simulink model "EVSystemConverterModel"  (R2024a)
settings: Solver=ode23t  StartTime=0.0  StopTime=0.08  RelTol=1e-3
libraries: fl_lib x16, nesl_utility x8, ee_lib x3, eePwmGenerator x3, batteryecm_lib x1
settings Model: Creator=callie  LastModifiedBy=callie
settings DataIOCC: ReturnWorkspaceOutputs=off
settings SimscapeCC: SimscapeLogType=all  SimscapeLogLimitData=off

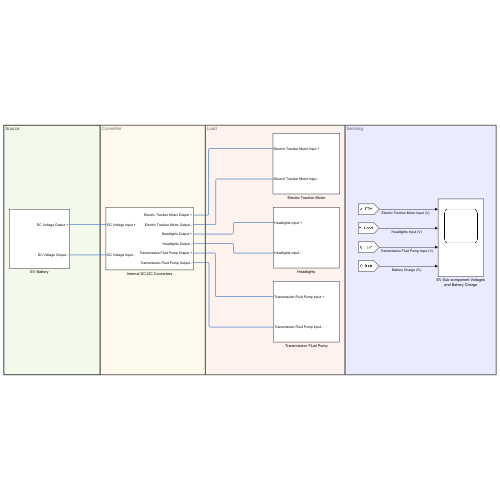
[thumbnail: Simulink's stored preview of the top-level diagram]
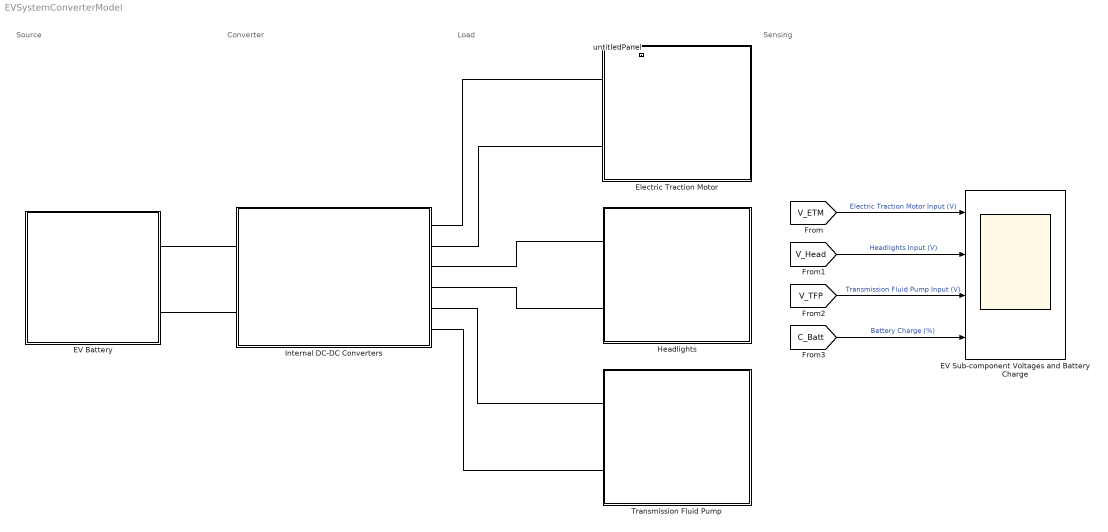
== system EVSystemConverterModel ==
  note: Sensing
  note: Load
  note: Converter
  note: Source
  EV Battery : Subsystem
      settings: PortSchema="{\"entries\":[{\"content\":{\"sides\":[{\"content\":{},\"type\":\"ConnectorPlacement.EquallySpacedRectSide\",\"uuid\":\"c6623932-9384-4505-9c8a-7aa7c6d03efe\"},{\"content\":{\"side\":\"RIGHT\"},\"type\":\"ConnectorPlacement.EquallySpacedRectSide\",\"uuid\":\"b63081fa-6f2e-4d52-89b7-0b15c2ff5a8a\"},{\"content\":{\"side\":\"TOP\"},\"type\":\"ConnectorPlacement.EquallySpacedRectSide\",\"uuid\":\"293a2b80-333e-46a9-baf9-140dd0ae167b\"},{\"content\":{\"connectorIds\":[\"RConn1\",\"RConn2\"],\"side\":\"BOTTOM\"},\"type\":\"ConnectorPlacement.EquallySpacedRectSide\",\"uuid\":\"5c4d294a-cecf-4357-a6de-56f8bde29aff\"}]},\"type\":\"ConnectorPlacement.EquallySpacedConnector\",\"uuid\":\"b1957f8b-46fc-490a-ae52-971fc17beee3\"}],\"packageUris\":[\"http://schema.mathworks.com/mf0/Connector/R2020b\"],\"version\":\"1.0\"}"
  EV Sub-component Voltages and Battery Charge : Scope  NumInputPorts=4
  Electric Traction Motor : Subsystem
      settings: PortSchema="{\"entries\":[{\"content\":{\"sides\":[{\"content\":{},\"type\":\"ConnectorPlacement.EquallySpacedRectSide\",\"uuid\":\"1c916003-081d-495c-ab06-e1419b6c539b\"},{\"content\":{\"side\":\"RIGHT\"},\"type\":\"ConnectorPlacement.EquallySpacedRectSide\",\"uuid\":\"f192687e-cae6-4b69-b15b-4d7b02c42b9f\"},{\"content\":{\"connectorIds\":[\"LConn1\",\"LConn2\"],\"side\":\"TOP\"},\"type\":\"ConnectorPlacement.EquallySpacedRectSide\",\"uuid\":\"4ee18eaf-a0eb-4206-a34f-c6cf4701fcf7\"}]},\"type\":\"ConnectorPlacement.EquallySpacedConnector\",\"uuid\":\"c4b359e2-4be8-4ef0-b2fa-d43323f3e4c6\"}],\"packageUris\":[\"http://schema.mathworks.com/mf0/Connector/R2020b\"],\"version\":\"1.0\"}"
  Headlights : Subsystem
      settings: PortSchema="{\"entries\":[{\"content\":{\"sides\":[{\"content\":{},\"type\":\"ConnectorPlacement.EquallySpacedRectSide\",\"uuid\":\"1c916003-081d-495c-ab06-e1419b6c539b\"},{\"content\":{\"side\":\"RIGHT\"},\"type\":\"ConnectorPlacement.EquallySpacedRectSide\",\"uuid\":\"f192687e-cae6-4b69-b15b-4d7b02c42b9f\"},{\"content\":{\"connectorIds\":[\"LConn1\",\"LConn2\"],\"side\":\"TOP\"},\"type\":\"ConnectorPlacement.EquallySpacedRectSide\",\"uuid\":\"4ee18eaf-a0eb-4206-a34f-c6cf4701fcf7\"}]},\"type\":\"ConnectorPlacement.EquallySpacedConnector\",\"uuid\":\"c4b359e2-4be8-4ef0-b2fa-d43323f3e4c6\"}],\"packageUris\":[\"http://schema.mathworks.com/mf0/Connector/R2020b\"],\"version\":\"1.0\"}"
  Internal DC-DC Converters : Subsystem
  Transmission Fluid Pump : Subsystem
      settings: PortSchema="{\"entries\":[{\"content\":{\"sides\":[{\"content\":{},\"type\":\"ConnectorPlacement.EquallySpacedRectSide\",\"uuid\":\"1c916003-081d-495c-ab06-e1419b6c539b\"},{\"content\":{\"side\":\"RIGHT\"},\"type\":\"ConnectorPlacement.EquallySpacedRectSide\",\"uuid\":\"f192687e-cae6-4b69-b15b-4d7b02c42b9f\"},{\"content\":{\"connectorIds\":[\"LConn1\",\"LConn2\"],\"side\":\"TOP\"},\"type\":\"ConnectorPlacement.EquallySpacedRectSide\",\"uuid\":\"4ee18eaf-a0eb-4206-a34f-c6cf4701fcf7\"}]},\"type\":\"ConnectorPlacement.EquallySpacedConnector\",\"uuid\":\"c4b359e2-4be8-4ef0-b2fa-d43323f3e4c6\"}],\"packageUris\":[\"http://schema.mathworks.com/mf0/Connector/R2020b\"],\"version\":\"1.0\"}"
  untitledPanel : Subsystem  Tag=HiddenForWebPanel  IsWebBlockPanel=on
  wires:
  [V_TFP] -> EV Sub-component Voltages and Battery Charge/3  "Transmission Fluid Pump Input (V)"
  [C_Batt] -> EV Sub-component Voltages and Battery Charge/4  "Battery Charge (%)"
  [V_Head] -> EV Sub-component Voltages and Battery Charge/2  "Headlights Input (V)"
  [V_ETM] -> EV Sub-component Voltages and Battery Charge/1  "Electric Traction Motor Input (V)"
  connections:
  EV Battery/RConn1 -- Internal DC-DC Converters/RConn1
  EV Battery/RConn2 -- Internal DC-DC Converters/RConn2
  Internal DC-DC Converters/LConn1 -- Electric Traction Motor/LConn1
  Internal DC-DC Converters/LConn2 -- Electric Traction Motor/LConn2
  Internal DC-DC Converters/LConn3 -- Headlights/LConn1
  Internal DC-DC Converters/LConn4 -- Headlights/LConn2
  Internal DC-DC Converters/LConn5 -- Transmission Fluid Pump/LConn1
  Transmission Fluid Pump/LConn2 -- Internal DC-DC Converters/LConn6

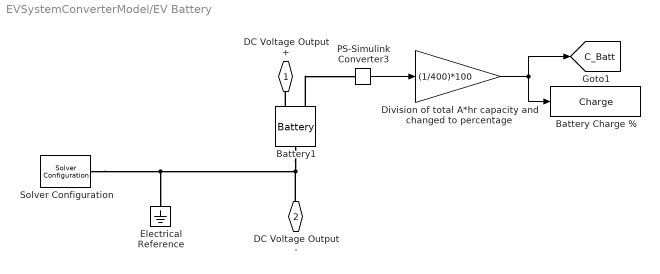
== system EVSystemConverterModel/EV Battery ==
  Battery Charge % : ToWorkspace  VariableName=Charge  SampleTime=-1
  Battery1 : batteryecm_lib/Battery  Vnom=350 V  prm_dir=simscape.enum.battery.prm_dir.disabled  R1_dis=2 Ohm  R1_ch=2 Ohm  R1=500 mOhm  prm_AH=simscape.enum.battery.prm_AH.finite  AH=400 A*hr  V1=290 V  AH1=331 A*hr  prm_R2=simscape.enum.battery.prm_R2.disabled  R2=2000 Ohm  Tmeas=298.15 K  charge_measurement_port=simscape.enum.battery.enable.yes  prm_dyn=simscape.enum.battery.prm_dyn.off  Rp1=0.005 Ohm  tau1=30 s  Rp2=0.005 Ohm  tau2=30 s  Rp3=0.005 Ohm  tau3=30 s  Rp4=0.005 Ohm  tau4=30 s  Rp5=0.005 Ohm  tau5=30 s  prm_fade=simscape.enum.battery.prm_fade.disabled  N_fade=100  AH_fade=45 A*hr  R1_fade=2.02 Ohm  R1_ch_fade=2.02 Ohm  V1_fade=10.35 V  prm_age=simscape.enum.battery.prm_age.disabled  prm_age_OCV=simscape.enum.battery.prm_age_OCV.OCV  OCV_age=0.9  SOC_age=60  Tmeas_age=298.15 K  delta_time_age_vec=[0] d  temperature_age_vec=[273] K  OCV_scaling_age=2.2134e6  OCV_offset_age=1.632e6  temp_exp_age=0.515833569 V  t_exp_age=0.75  Vnom_T2=12 V  R1_T2=2.2 Ohm  R1_T2_dis=2.2 Ohm  R1_T2_ch=2.2 Ohm  V1_T2=11.4 V  R2_T2=2200 Ohm  Rp1_T2=0.005 Ohm  tau1_T2=30 s  Rp2_T2=0.005 Ohm  tau2_T2=30 s  Rp3_T2=0.005 Ohm  tau3_T2=30 s  Rp4_T2=0.005 Ohm  tau4_T2=30 s  Rp5_T2=0.005 Ohm  tau5_T2=30 s  Tmeas2=273.15 K  thermal_port=simscape.enum.thermaleffects.omit  thermal_mass=30000 J/K  i_specify=off  i_priority=None  i=0 A  i_nominal_specify=off  i_nominal_value=1  i_nominal_unit=A  v_specify=on  v_priority=None  v=350 V  v_nominal_specify=off  v_nominal_value=22.8  v_nominal_unit=V  charge_specify=on  charge_priority=High  charge=400 A*hr  charge_nominal_specify=on  charge_nominal_value=2.3  charge_nominal_unit=A*hr  num_cycles_specify=off  num_cycles_priority=High  num_cycles=0  num_cycles_nominal_specify=off  num_cycles_nominal_value=1  num_cycles_nominal_unit=1  temperature_specify=off  temperature_priority=High  temperature=298.15 K  temperature_nominal_specify=off  temperature_nominal_value=1  temperature_nominal_unit=K
      settings: LibrarySourceBlock=batt_lib/Cells/Battery  InternalSimscapePortConfiguration="{\"Bottom\":[],\"Left\":[{\"id\":\"p\",\"label\":\"+\",\"type\":\"foundation.electrical.electrical\"},{\"id\":\"q\",\"label\":\"q\",\"type\":\"output\"}],\"Right\":[{\"id\":\"n\",\"label\":\"-\",\"type\":\"foundation.electrical.electrical\"}],\"Top\":[]}"
  Division of total A*hr capacity and changed to percentage : Gain  Gain=(1/400)*100
  Electrical Reference : fl_lib/Electrical/Electrical Elements/Electrical Reference
  PS-Simulink Converter3 : nesl_utility/PS-Simulink Converter  PhysicalDomain=network_engine_domain  SubClassName=ps_output  LeftPortType=input  RightPortType=output  PseudoPeriodic=off  Frequencies=[]  VectorFormat=inherit  Unit=A*hr  AffineConversion=off
  Solver Configuration : nesl_utility/Solver Configuration  PhysicalDomain=network_engine_domain  SubClassName=solver  LeftPortType=input  RightPortType=generic  Tones=[]  Harmonics=[]  SimulateNoise=off  Profile=off  UseLocalSampling=off  EnableSwitchedLinearOptims=on  FrequencyDomain=off  UseCCode=off  RelTol=0.001  AbsTol=1e-06  MinStep=1e-09  ToWorkspace=off  RevertToSquareIcSolve=off  NumHomotopyIterations=100  PhasorMode=off  PhasorModeNumHarmonics=1  ConsistencySolver=NEWTON_FTOL  IndexReductionMethod=DerivativeReplacement  DoDC=off  ResidualTolerance=1e-09  ConsistencyTolSource=GLOBAL  ConsistencyAbsTol=0.001  ConsistencyRelTol=0.001  ConsistencyTolFactor=0.001  UseLocalSolver=off  LocalSolverChoice=NE_BACKWARD_EULER_ADVANCER  ResolveIndetEquations=on  FunctionEvalNumThread=1  LocalSolverSampleTime=0.00001  DoFixedCost=off  MaxNonlinIter=3  MaxModeIter=2  ComputeImpulses=off  ImpulseIterations=2  LinearAlgebra=auto  LinearAlgebraNumThread=0  EquationFormulation=NE_TIME_EF  DelaysMemoryBudget=1024  AutomaticFiltering=on  FilteringTimeConstant=0.001  PartitionStorageMethod=AS_NEEDED  PartitionMemoryBudget=1024  PartitionMethod=ROBUST  MultibodyUseLocalSolver=off  MultibodyLocalSolverChoice=ODE1  MultibodyLocalSolverSampleTime=0.001
  DC Voltage Output + : PMIOPort  Side=Right
  DC Voltage Output - : PMIOPort  Port=2  Side=Right
  tag scope: C_Batt=global
  wires:
  Division of total A*hr capacity and changed to percentage/1 -> [C_Batt], Battery Charge %/1
  PS-Simulink Converter3/1 -> Division of total A*hr capacity and changed to percentage/1
  connections:
  Solver Configuration/RConn1 -- Battery1/RConn1 -- DC Voltage Output -/RConn1 -- Electrical Reference/LConn1
  Battery1/LConn1 -- DC Voltage Output +/RConn1
  Battery1/LConn2 -- PS-Simulink Converter3/LConn1

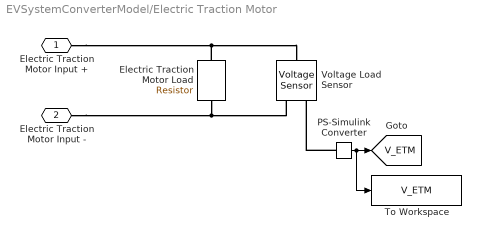
== system EVSystemConverterModel/Electric Traction Motor ==
  Electric Traction Motor Load : fl_lib/Electrical/Electrical Elements/Resistor  R=3 Ohm  i_specify=off  i_priority=High  i=0 A  i_nominal_specify=off  i_nominal_value=1  i_nominal_unit=A  v_specify=off  v_priority=High  v=0 V  v_nominal_specify=off  v_nominal_value=1  v_nominal_unit=V
  PS-Simulink Converter : nesl_utility/PS-Simulink Converter  PhysicalDomain=network_engine_domain  SubClassName=ps_output  LeftPortType=input  RightPortType=output  PseudoPeriodic=off  Frequencies=[]  VectorFormat=inherit  Unit=V  AffineConversion=off
  To Workspace : ToWorkspace  VariableName=V_ETM  SampleTime=-1
  Voltage Load Sensor : fl_lib/Electrical/Electrical Sensors/Voltage Sensor
  Electric Traction Motor Input + : PMIOPort  Side=Left
  Electric Traction Motor Input - : PMIOPort  Port=2  Side=Left
  tag scope: V_ETM=global
  wires:
  PS-Simulink Converter/1 -> To Workspace/1, [V_ETM]
  connections:
  Electric Traction Motor Input -/RConn1 -- Electric Traction Motor Load/RConn1 -- Voltage Load Sensor/RConn2
  Electric Traction Motor Input +/RConn1 -- Electric Traction Motor Load/LConn1 -- Voltage Load Sensor/LConn1
  PS-Simulink Converter/LConn1 -- Voltage Load Sensor/RConn1

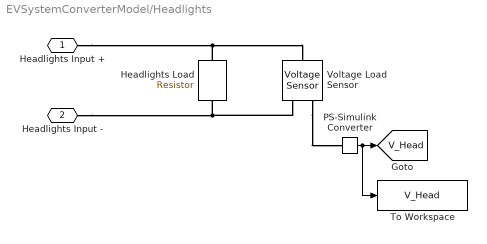
== system EVSystemConverterModel/Headlights ==
  Headlights Load : fl_lib/Electrical/Electrical Elements/Resistor  R=20 Ohm  i_specify=off  i_priority=High  i=0 A  i_nominal_specify=off  i_nominal_value=1  i_nominal_unit=A  v_specify=off  v_priority=High  v=0 V  v_nominal_specify=off  v_nominal_value=1  v_nominal_unit=V
  PS-Simulink Converter : nesl_utility/PS-Simulink Converter  PhysicalDomain=network_engine_domain  SubClassName=ps_output  LeftPortType=input  RightPortType=output  PseudoPeriodic=off  Frequencies=[]  VectorFormat=inherit  Unit=V  AffineConversion=off
  To Workspace : ToWorkspace  VariableName=V_Head  SampleTime=-1
  Voltage Load Sensor : fl_lib/Electrical/Electrical Sensors/Voltage Sensor
  Headlights Input + : PMIOPort  Side=Left
  Headlights Input - : PMIOPort  Port=2  Side=Left
  tag scope: V_Head=global
  wires:
  PS-Simulink Converter/1 -> To Workspace/1, [V_Head]
  connections:
  Headlights Load/LConn1 -- Headlights Input +/RConn1 -- Voltage Load Sensor/LConn1
  Voltage Load Sensor/RConn2 -- Headlights Input -/RConn1 -- Headlights Load/RConn1
  Voltage Load Sensor/RConn1 -- PS-Simulink Converter/LConn1

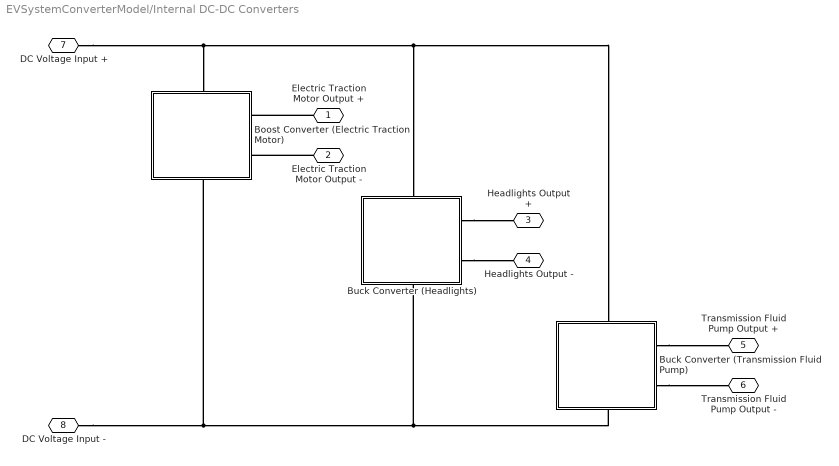
== system EVSystemConverterModel/Internal DC-DC Converters ==
  "Boost Converter (Electric Traction Motor)  " : Subsystem
      settings: PortSchema="{\"entries\":[{\"content\":{\"sides\":[{\"content\":{},\"type\":\"ConnectorPlacement.EquallySpacedRectSide\",\"uuid\":\"de7f9f94-85d7-4c11-a379-f82d9a676ef7\"},{\"content\":{\"connectorIds\":[\"RConn1\",\"RConn2\"],\"side\":\"RIGHT\"},\"type\":\"ConnectorPlacement.EquallySpacedRectSide\",\"uuid\":\"401d076f-92b5-441a-942d-9f536a3912de\"},{\"content\":{\"connectorIds\":[\"LConn1\"],\"side\":\"TOP\"},\"type\":\"ConnectorPlacement.EquallySpacedRectSide\",\"uuid\":\"060ca2a1-5903-409e-b252-71c13fd12de7\"},{\"content\":{\"connectorIds\":[\"RConn3\"],\"side\":\"BOTTOM\"},\"type\":\"ConnectorPlacement.EquallySpacedRectSide\",\"uuid\":\"bdbe130f-4b5d-4c03-bda1-a69c86499370\"}]},\"type\":\"ConnectorPlacement.EquallySpacedConnector\",\"uuid\":\"c546e283-911b-4991-8697-f1e295eb6532\"}],\"packageUris\":[\"http://schema.mathworks.com/mf0/Connector/R2020b\"],\"version\":\"1.0\"}"
  "Buck Converter (Transmission Fluid Pump)  " : Subsystem
      settings: PortSchema="{\"entries\":[{\"content\":{\"sides\":[{\"content\":{},\"type\":\"ConnectorPlacement.EquallySpacedRectSide\",\"uuid\":\"de7f9f94-85d7-4c11-a379-f82d9a676ef7\"},{\"content\":{\"connectorIds\":[\"RConn1\",\"RConn2\"],\"side\":\"RIGHT\"},\"type\":\"ConnectorPlacement.EquallySpacedRectSide\",\"uuid\":\"401d076f-92b5-441a-942d-9f536a3912de\"},{\"content\":{\"connectorIds\":[\"LConn1\"],\"side\":\"TOP\"},\"type\":\"ConnectorPlacement.EquallySpacedRectSide\",\"uuid\":\"060ca2a1-5903-409e-b252-71c13fd12de7\"},{\"content\":{\"connectorIds\":[\"RConn3\"],\"side\":\"BOTTOM\"},\"type\":\"ConnectorPlacement.EquallySpacedRectSide\",\"uuid\":\"bdbe130f-4b5d-4c03-bda1-a69c86499370\"}]},\"type\":\"ConnectorPlacement.EquallySpacedConnector\",\"uuid\":\"c546e283-911b-4991-8697-f1e295eb6532\"}],\"packageUris\":[\"http://schema.mathworks.com/mf0/Connector/R2020b\"],\"version\":\"1.0\"}"
  "Buck Converter (Headlights)  " : Subsystem
      settings: PortSchema="{\"entries\":[{\"content\":{\"sides\":[{\"content\":{},\"type\":\"ConnectorPlacement.EquallySpacedRectSide\",\"uuid\":\"de7f9f94-85d7-4c11-a379-f82d9a676ef7\"},{\"content\":{\"connectorIds\":[\"RConn1\",\"RConn2\"],\"side\":\"RIGHT\"},\"type\":\"ConnectorPlacement.EquallySpacedRectSide\",\"uuid\":\"401d076f-92b5-441a-942d-9f536a3912de\"},{\"content\":{\"connectorIds\":[\"LConn1\"],\"side\":\"TOP\"},\"type\":\"ConnectorPlacement.EquallySpacedRectSide\",\"uuid\":\"060ca2a1-5903-409e-b252-71c13fd12de7\"},{\"content\":{\"connectorIds\":[\"RConn3\"],\"side\":\"BOTTOM\"},\"type\":\"ConnectorPlacement.EquallySpacedRectSide\",\"uuid\":\"bdbe130f-4b5d-4c03-bda1-a69c86499370\"}]},\"type\":\"ConnectorPlacement.EquallySpacedConnector\",\"uuid\":\"c546e283-911b-4991-8697-f1e295eb6532\"}],\"packageUris\":[\"http://schema.mathworks.com/mf0/Connector/R2020b\"],\"version\":\"1.0\"}"
  Electric Traction Motor Output + : PMIOPort  Side=Left
  Electric Traction Motor Output - : PMIOPort  Port=2  Side=Left
  Headlights Output + : PMIOPort  Port=3  Side=Left
  Headlights Output - : PMIOPort  Port=4  Side=Left
  Transmission Fluid Pump Output + : PMIOPort  Port=5  Side=Left
  Transmission Fluid Pump Output - : PMIOPort  Port=6  Side=Left
  DC Voltage Input + : PMIOPort  Port=7  Side=Right
  DC Voltage Input - : PMIOPort  Port=8  Side=Right
  connections:
  DC Voltage Input +/RConn1 -- "Buck Converter (Transmission Fluid Pump)  "/LConn1 -- "Buck Converter (Headlights)  "/LConn1 -- "Boost Converter (Electric Traction Motor)  "/LConn1
  DC Voltage Input -/RConn1 -- "Boost Converter (Electric Traction Motor)  "/RConn3 -- "Buck Converter (Transmission Fluid Pump)  "/RConn3 -- "Buck Converter (Headlights)  "/RConn3
  Electric Traction Motor Output +/RConn1 -- "Boost Converter (Electric Traction Motor)  "/RConn1
  Electric Traction Motor Output -/RConn1 -- "Boost Converter (Electric Traction Motor)  "/RConn2
  "Buck Converter (Headlights)  "/RConn1 -- Headlights Output +/RConn1
  "Buck Converter (Headlights)  "/RConn2 -- Headlights Output -/RConn1
  "Buck Converter (Transmission Fluid Pump)  "/RConn1 -- Transmission Fluid Pump Output +/RConn1
  "Buck Converter (Transmission Fluid Pump)  "/RConn2 -- Transmission Fluid Pump Output -/RConn1

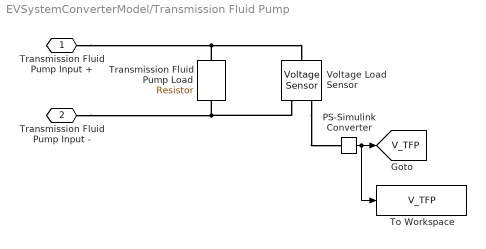
== system EVSystemConverterModel/Transmission Fluid Pump ==
  PS-Simulink Converter : nesl_utility/PS-Simulink Converter  PhysicalDomain=network_engine_domain  SubClassName=ps_output  LeftPortType=input  RightPortType=output  PseudoPeriodic=off  Frequencies=[]  VectorFormat=inherit  Unit=V  AffineConversion=off
  To Workspace : ToWorkspace  VariableName=V_TFP  SampleTime=-1
  Transmission Fluid Pump Load : fl_lib/Electrical/Electrical Elements/Resistor  R=40 Ohm  i_specify=off  i_priority=High  i=0 A  i_nominal_specify=off  i_nominal_value=1  i_nominal_unit=A  v_specify=off  v_priority=High  v=0 V  v_nominal_specify=off  v_nominal_value=1  v_nominal_unit=V
  Voltage Load Sensor : fl_lib/Electrical/Electrical Sensors/Voltage Sensor
  Transmission Fluid Pump Input + : PMIOPort  Side=Left
  Transmission Fluid Pump Input - : PMIOPort  Port=2  Side=Left
  tag scope: V_TFP=global
  wires:
  PS-Simulink Converter/1 -> To Workspace/1, [V_TFP]
  connections:
  Transmission Fluid Pump Load/LConn1 -- Transmission Fluid Pump Input +/RConn1 -- Voltage Load Sensor/LConn1
  Voltage Load Sensor/RConn2 -- Transmission Fluid Pump Input -/RConn1 -- Transmission Fluid Pump Load/RConn1
  Voltage Load Sensor/RConn1 -- PS-Simulink Converter/LConn1

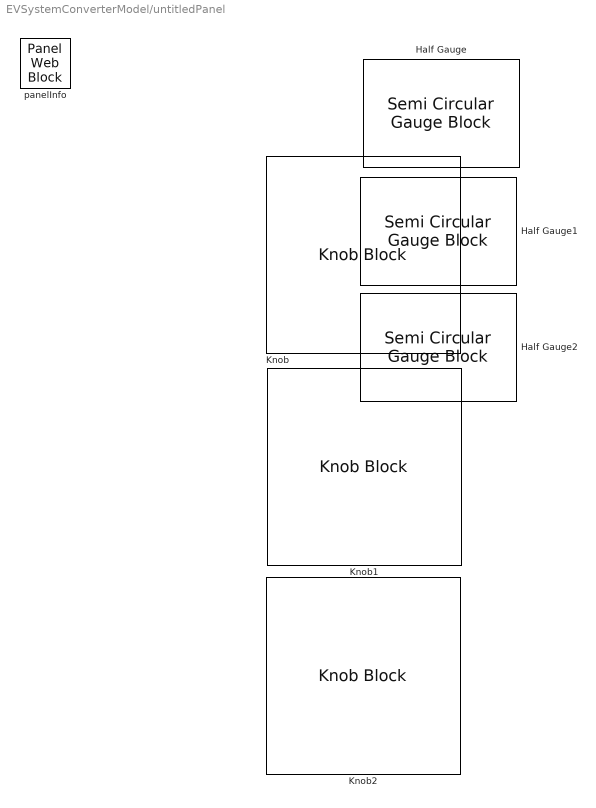
== system EVSystemConverterModel/untitledPanel ==
  Half Gauge : SemiCircularGaugeBlock  Tag=HiddenForWebPanel  PanelInfo="{\"height\":179,\"left\":517,\"panelId\":\"panelId-d2794712-f72d-43ac-b620-292c36f24508\",\"top\":127,\"type\":\"panelChild\",\"version\":\"2019b\",\"width\":257,\"zIndex\":1500008}"  LabelPosition=Hide  ScaleMax=500  TickInterval=100
  Half Gauge1 : SemiCircularGaugeBlock  Tag=HiddenForWebPanel  PanelInfo="{\"height\":179,\"left\":520,\"panelId\":\"panelId-d2794712-f72d-43ac-b620-292c36f24508\",\"top\":335,\"type\":\"panelChild\",\"version\":\"2019b\",\"width\":257,\"zIndex\":1500010}"  LabelPosition=Hide  ScaleMax=24  TickInterval=4
  Half Gauge2 : SemiCircularGaugeBlock  Tag=HiddenForWebPanel  PanelInfo="{\"height\":179,\"left\":522,\"panelId\":\"panelId-d2794712-f72d-43ac-b620-292c36f24508\",\"top\":542,\"type\":\"panelChild\",\"version\":\"2019b\",\"width\":257,\"zIndex\":1500012}"  LabelPosition=Hide  ScaleMax=24  TickInterval=4
  Knob : KnobBlock  Tag=HiddenForWebPanel  PanelInfo="{\"height\":197,\"left\":250,\"panelId\":\"panelId-d2794712-f72d-43ac-b620-292c36f24508\",\"top\":123,\"type\":\"panelChild\",\"version\":\"2019b\",\"width\":188,\"zIndex\":1500014}"  LabelPosition=Hide
  Knob1 : KnobBlock  Tag=HiddenForWebPanel  PanelInfo="{\"height\":192,\"left\":251,\"panelId\":\"panelId-d2794712-f72d-43ac-b620-292c36f24508\",\"top\":335,\"type\":\"panelChild\",\"version\":\"2019b\",\"width\":189,\"zIndex\":1500016}"  LabelPosition=Hide
  Knob2 : KnobBlock  Tag=HiddenForWebPanel  PanelInfo="{\"height\":192,\"left\":250,\"panelId\":\"panelId-d2794712-f72d-43ac-b620-292c36f24508\",\"top\":540,\"type\":\"panelChild\",\"version\":\"2019b\",\"width\":189,\"zIndex\":1500018}"  LabelPosition=Hide
  panelInfo : PanelWebBlock  Tag=HiddenForWebPanel  PanelInfo="{\"compacted\":false,\"height\":736,\"isActiveTab\":true,\"labels\":{\"label0978741734\":{\"deleted\":false,\"left\":11,\"settings\":{\"backgroundColor\":\"rgba(0, 0, 0, 0)\",\"bold\":false,\"font\":\"Arial\",\"fontColor\":\"black\",\"fontSize\":1.5,\"italicized\":false,\"underlined\":false},\"text\":\"Duty Cycle Control Panel\",\"top\":21},\"label3712848784\":{\"deleted\":false,\"left\":28,\"settings\":{\"backgroundColor\":\"rgba(0, 0, 0, 0)\",\"bold\":false,\"font\":\"Arial\",\"fontColor\":\"black\",\"fontSize\":1.5,\"italicized\":false,\"underlined\":false},\"text\":\"Headlights\",\"top\":416},\"label5155327209\":{\"deleted\":false,\"left\":44,\"settings\":{\"backgroundColor\":\"rgba(0, 0, 0, 0)\",\"bold\":false,\"font\":\"Arial\",\"fontColor\":\"black\",\"fontSize\":1.5,\"italicized\":false,\"underlined\":false},\"text\":\"Electric\",\"top\":175},\"label6478120002\":{\"deleted\":false,\"left\":14,\"settings\":{\"backgroundColor\":\"rgba(0, 0, 0, 0)\",\"bold\":false,\"font\":\"Arial\",\"fontColor\":\"black\",\"fontSize\":1.53,\"italicized\":false,\"underlined\":false},\"text\":\"Traction Motor\",\"top\":215},\"label7159950870\":{\"deleted\":false,\"left\":30,\"settings\":{\"backgroundColor\":\"rgba(0, 0, 0, 0)\",\"bold\":false,\"font\":\"Arial\",\"fontColor\":\"black\",\"fontSize\":1.53,\"italicized\":false,\"underlined\":false},\"text\":\"Fluid Pump\",\"top\":638},\"label7400305898\":{\"deleted\":false,\"left\":223,\"settings\":{\"backgroundColor\":\"rgba(0, 0, 0, 0)\",\"bold\":false,\"font\":\"Arial\",\"fontColor\":\"black\",\"fontSize\":1.38,\"italicized\":false,\"underlined\":false},\"text\":\"Duty Cycle Percentage\",\"top\":85},\"label8434406955\":{\"deleted\":false,\"left\":482,\"settings\":{\"backgroundColor\":\"rgba(0, 0, 0, 0)\",\"bold\":false,\"font\":\"Arial\",\"fontColor\":\"black\",\"fontSize\":1.38,\"italicized\":false,\"underlined\":false},\"text\":\"Sub-component Voltage Reading\",\"top\":84},\"label9519776243\":{\"deleted\":false,\"left\":14,\"settings\":{\"backgroundColor\":\"rgba(0, 0, 0, 0)\",\"bold\":false,\"font\":\"Arial\",\"fontColor\":\"black\",\"fontSize\":1.64,\"italicized\":false,\"underlined\":false},\"text\":\"Transmission\",\"top\":608}},\"left\":898,\"name\":\"Panel\",\"panelId\":\"panelId-d2794712-f72d-43ac-b620-292c36f24508\",\"popoutData\":{\"height\":0,\"left\":0,\"maximized\":false,\"top\":0,\"width\":0},\"popoutMode\":\"component\",\"tabIndex\":0,\"tabbedSetId\":\"tabbedSet3198299715\",\"top\":68,\"type\":\"panel\",\"version\":\"2019b\",\"visible\":true,\"width\":818,\"zIndex\":1500002}"  PanelSnapshot=<binary blob, 58640 chars, not shown>

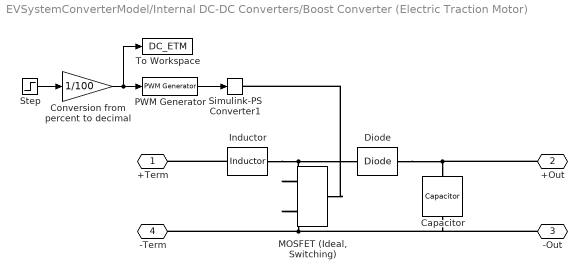
== system EVSystemConverterModel/Internal DC-DC Converters/Boost Converter (Electric Traction Motor)   ==
  Capacitor : fl_lib/Electrical/Electrical Elements/Capacitor  c=5e-4 F  r=1e-6 Ohm  g=0 1/Ohm  i_specify=off  i_priority=None  i=0 A  i_nominal_specify=off  i_nominal_value=1  i_nominal_unit=A  v_specify=off  v_priority=None  v=0 V  v_nominal_specify=off  v_nominal_value=1  v_nominal_unit=V  vc_specify=off  vc_priority=High  vc=0 V  vc_nominal_specify=off  vc_nominal_value=1  vc_nominal_unit=V
  Conversion from percent to decimal : Gain  Gain=1/100
  Diode : fl_lib/Electrical/Electrical Elements/Diode  Vf=0.6 V  Ron=1e-3 Ohm  Goff=1e-08 1/Ohm  i_specify=off  i_priority=High  i=0 A  i_nominal_specify=off  i_nominal_value=1  i_nominal_unit=A  v_specify=off  v_priority=High  v=0 V  v_nominal_specify=off  v_nominal_value=1  v_nominal_unit=V
  Inductor : fl_lib/Electrical/Electrical Elements/Inductor  l=10e-3 H  r=0 Ohm  g=1e-9 1/Ohm  i_specify=off  i_priority=None  i=0 A  i_nominal_specify=off  i_nominal_value=1  i_nominal_unit=A  v_specify=off  v_priority=None  v=0 V  v_nominal_specify=off  v_nominal_value=1  v_nominal_unit=V  i_L_specify=off  i_L_priority=High  i_L=0 A  i_L_nominal_specify=off  i_L_nominal_value=1  i_L_nominal_unit=A
  "MOSFET (Ideal, Switching)" : ee_lib/Semiconductors & Converters/MOSFET (Ideal, Switching)  port_option=ee.enum.controlport.ps  Rds=1e-3 Ohm  Goff=1e-6 1/Ohm  Vth=0.1 V  diode_param=ee.enum.semiconductors.protectionDiode.external  diode_Vf=0.6 V  diode_Ron=1e-3 Ohm  diode_Goff=1e-5 1/Ohm  diode_C=50e-9 F  diode_iRM=-235 A  diode_iF=300 A  diode_idot=-50 A/us  diode_trr_param=ee.enum.converters.diodeReverseParam.trr_factor  diode_trr_factor=3  diode_trr=15 us  diode_Qrr=1500 s*uA  ids_specify=off  ids_priority=None  ids=0 A  ids_nominal_specify=off  ids_nominal_value=1  ids_nominal_unit=A  vds_specify=off  vds_priority=None  vds=0 V  vds_nominal_specify=off  vds_nominal_value=1  vds_nominal_unit=V  vgs_specify=off  vgs_priority=None  vgs=0 V  vgs_nominal_specify=off  vgs_nominal_value=1  vgs_nominal_unit=V  thermal_loss_option=ee.enum.converters.thermalLossOption.constantvalues  Von_data=[0, 1.8, 3.2, 6, 10, 16; 0, 2, 5.5, 9.5, 15, 25] V  Tj=[298.15, 448.15] K  Iout_data=[0, 20, 40, 60, 80, 100] A  Eon_data=[0, 55.04, 124.57, 235.53, 362.12; 0, 71.25, 161.25, 304.88, 468.75] * 1e-6 J  Eoff_data=[0, 18, 30, 56.1, 76.5; 0, 22.5, 37.5, 70.13, 95.63] * 1e-6 J  Eon_data_3D=[zeros(2, 5, 3)] J  Eoff_data_3D=[zeros(2, 5, 3)] J  Tj_loss=[298.15, 448.15] K  Iout_data_loss=[0, 10, 20, 30, 40] A  tabulateWithVds=false  Vds_loss=[0, 150, 300] V  Eon_scalar=22.86e-3 J  Eoff_scalar=17.14e-3 J  Voff=300 V  Iout_scalar=600 A  useCurrentFromPreviousCycle=false  useVoltageFromPreviousCycle=false  diodeModelType=ee.enum.converters.diodeModelType.pwl  diodeTableType=ee.enum.diode.tableType.IfMat  diode_ReverseIVType=ee.enum.diode.diodeReverseIV.constant  diode_IfMat=[.07, .12, .19, 1.75, 4.24, 7.32, 11.2; .16, .3, .72, 2.14, 4.02, 6.35, 9.12] A  diode_VfMat=[.9, 1.15, 1.25, 1.5, 1.75, 2.17, 2.6, 2.85; .58, .68, .75, 1.1, 1.38, 1.77, 2.27, 2.7] V  diode_TjVec=[25, 125] degC  diode_VfVec=[.5, .7, .9, 1.3, 1.7, 2.1, 2.5] V  diode_IfVec=[.1, .2, .5, 1, 2, 4, 7, 10] A  diode_IrMat=[1e-06, 2e-06, 5e-06, 1e-05, 2.5e-05, 5e-05, .0001; 2e-06, 5e-06, 1e-05, 4e-05, 8e-05, .0002, .0005] A  diode_VrMat=[10, 100, 200, 250, 300, 325, 350; 10, 70, 160, 220, 270, 300, 320] V  diode_VrVec=[10, 20, 40, 50, 70, 80, 100] V  diode_IrVec=[1e-06, 2e-06, 5e-06, 1e-05, 2e-05, 5e-05, .0001] A  diode_Vr=-600 V  diode_Ls=150 nH  diode_Erec=0.03 J  diode_rec_loss_model=ee.enum.diode.reverseRecoveryModel.fixed  diode_ErecVal=0 J  diode_scaleWithIandV=true  diode_ErecMat=zeros(2, 3) J  diode_TjrecVec=[298.15, 398.15] K  diode_IfrecVec=[.1, 1, 10] A  diode_IrecVal=10 A  diode_VrecVal=10 V  diode_tFilter=1 / 1000 / 100 s  thermal_network_parameterization=ee.enum.thermalNetworkTopology.external  Rth=[.03, .2] K/W  Rth_Cauer=[.03, .1, .2] K/W  Rth_Foster=[.03, .2] K/W  thermal_mass_parameterization=ee.enum.thermalNetwork.timeconstant  thermal_mass=[3, 25] J/K  thermal_mass_Cauer=[3, 10, 25] J/K  thermal_mass_Foster=[33, 50] J/K  thermal_time_constant=[.1, 5] s  thermal_time_constant_Cauer=[.1, 1, 5] s  thermal_time_constant_Foster=[1, 10] s  thermal_mass_initial_temperatures=[25, 25] degC  thermal_mass_initial_temperatures_Cauer=[25, 25, 25] degC  junction_thermal_mass=0.1 J/K  Tvec_initial_Foster=[25, 25, 25, 25] degC  no_thermal_network=0  junction_temperature_specify=off  junction_temperature_priority=None  junction_temperature=25 degC  junction_temperature_nominal_specify=off  junction_temperature_nominal_value=1  junction_temperature_nominal_unit=degC  Qj_specify=off  Qj_priority=None  Qj=0 W  Qj_nominal_specify=off  Qj_nominal_value=1  Qj_nominal_unit=W  accumulatedSwitchingLosses_specify=off  accumulatedSwitchingLosses_priority=None  accumulatedSwitchingLosses=0 J
  PWM Generator : eePwmGenerator/PWM Generator  CarrCount=Up  Tper=1/10000  Tdelay=0  Ts=0
  Simulink-PS Converter1 : nesl_utility/Simulink-PS Converter  PhysicalDomain=network_engine_domain  SubClassName=ps_input  LeftPortType=input  RightPortType=output  PseudoPeriodic=off  Frequencies=[]  NoiseDistribution=none  NoiseParameters=[]  Unit=V  AffineConversion=off  FilteringAndDerivatives=provide  SimscapeFilterOrder=1  InputFilterTimeConstant=0.001  UdotUserProvided=0
  Step : Step  Time=0.035  After=0  SampleTime=0
  To Workspace : ToWorkspace  VariableName=DC_ETM  SampleTime=-1
  +Term : PMIOPort  Side=Left
  +Out : PMIOPort  Port=2  Side=Right
  -Out : PMIOPort  Port=3  Side=Right
  -Term : PMIOPort  Port=4  Side=Right
  wires:
  Step/1 -> Conversion from percent to decimal/1
  PWM Generator/1 -> Simulink-PS Converter1/1
  Conversion from percent to decimal/1 -> To Workspace/1, PWM Generator/1
  connections:
  +Out/RConn1 -- Diode/RConn1 -- Capacitor/LConn1
  -Out/RConn1 -- Capacitor/RConn1 -- -Term/RConn1 -- "MOSFET (Ideal, Switching)"/RConn2
  "MOSFET (Ideal, Switching)"/LConn1 -- Simulink-PS Converter1/RConn1
  Inductor/LConn1 -- +Term/RConn1
  Inductor/RConn1 -- "MOSFET (Ideal, Switching)"/RConn1 -- Diode/LConn1

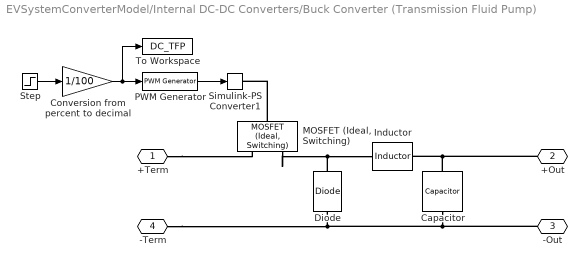
== system EVSystemConverterModel/Internal DC-DC Converters/Buck Converter (Transmission Fluid Pump)   ==
  Capacitor : fl_lib/Electrical/Electrical Elements/Capacitor  c=3e-6 F  r=1e-6 Ohm  g=0 1/Ohm  i_specify=off  i_priority=None  i=0 A  i_nominal_specify=off  i_nominal_value=1  i_nominal_unit=A  v_specify=off  v_priority=None  v=0 V  v_nominal_specify=off  v_nominal_value=1  v_nominal_unit=V  vc_specify=off  vc_priority=High  vc=0 V  vc_nominal_specify=off  vc_nominal_value=1  vc_nominal_unit=V
  Conversion from percent to decimal : Gain  Gain=1/100
  Diode : fl_lib/Electrical/Electrical Elements/Diode  Vf=0.6 V  Ron=1e-3 Ohm  Goff=1e-08 1/Ohm  i_specify=off  i_priority=High  i=0 A  i_nominal_specify=off  i_nominal_value=1  i_nominal_unit=A  v_specify=off  v_priority=High  v=0 V  v_nominal_specify=off  v_nominal_value=1  v_nominal_unit=V
  Inductor : fl_lib/Electrical/Electrical Elements/Inductor  l=8e-3 H  r=0 Ohm  g=1e-9 1/Ohm  i_specify=off  i_priority=None  i=0 A  i_nominal_specify=off  i_nominal_value=1  i_nominal_unit=A  v_specify=off  v_priority=None  v=0 V  v_nominal_specify=off  v_nominal_value=1  v_nominal_unit=V  i_L_specify=off  i_L_priority=High  i_L=0 A  i_L_nominal_specify=off  i_L_nominal_value=1  i_L_nominal_unit=A
  "MOSFET (Ideal, Switching)" : ee_lib/Semiconductors & Converters/MOSFET (Ideal, Switching)  port_option=ee.enum.controlport.ps  Rds=1e-3 Ohm  Goff=1e-6 1/Ohm  Vth=0.1 V  diode_param=ee.enum.semiconductors.protectionDiode.external  diode_Vf=0.6 V  diode_Ron=1e-3 Ohm  diode_Goff=1e-5 1/Ohm  diode_C=50e-9 F  diode_iRM=-235 A  diode_iF=300 A  diode_idot=-50 A/us  diode_trr_param=ee.enum.converters.diodeReverseParam.trr_factor  diode_trr_factor=3  diode_trr=15 us  diode_Qrr=1500 s*uA  ids_specify=off  ids_priority=None  ids=0 A  ids_nominal_specify=off  ids_nominal_value=1  ids_nominal_unit=A  vds_specify=off  vds_priority=None  vds=0 V  vds_nominal_specify=off  vds_nominal_value=1  vds_nominal_unit=V  vgs_specify=off  vgs_priority=None  vgs=0 V  vgs_nominal_specify=off  vgs_nominal_value=1  vgs_nominal_unit=V  thermal_loss_option=ee.enum.converters.thermalLossOption.constantvalues  Von_data=[0, 1.8, 3.2, 6, 10, 16; 0, 2, 5.5, 9.5, 15, 25] V  Tj=[298.15, 448.15] K  Iout_data=[0, 20, 40, 60, 80, 100] A  Eon_data=[0, 55.04, 124.57, 235.53, 362.12; 0, 71.25, 161.25, 304.88, 468.75] * 1e-6 J  Eoff_data=[0, 18, 30, 56.1, 76.5; 0, 22.5, 37.5, 70.13, 95.63] * 1e-6 J  Eon_data_3D=[zeros(2, 5, 3)] J  Eoff_data_3D=[zeros(2, 5, 3)] J  Tj_loss=[298.15, 448.15] K  Iout_data_loss=[0, 10, 20, 30, 40] A  tabulateWithVds=false  Vds_loss=[0, 150, 300] V  Eon_scalar=22.86e-3 J  Eoff_scalar=17.14e-3 J  Voff=300 V  Iout_scalar=600 A  useCurrentFromPreviousCycle=false  useVoltageFromPreviousCycle=false  diodeModelType=ee.enum.converters.diodeModelType.pwl  diodeTableType=ee.enum.diode.tableType.IfMat  diode_ReverseIVType=ee.enum.diode.diodeReverseIV.constant  diode_IfMat=[.07, .12, .19, 1.75, 4.24, 7.32, 11.2; .16, .3, .72, 2.14, 4.02, 6.35, 9.12] A  diode_VfMat=[.9, 1.15, 1.25, 1.5, 1.75, 2.17, 2.6, 2.85; .58, .68, .75, 1.1, 1.38, 1.77, 2.27, 2.7] V  diode_TjVec=[25, 125] degC  diode_VfVec=[.5, .7, .9, 1.3, 1.7, 2.1, 2.5] V  diode_IfVec=[.1, .2, .5, 1, 2, 4, 7, 10] A  diode_IrMat=[1e-06, 2e-06, 5e-06, 1e-05, 2.5e-05, 5e-05, .0001; 2e-06, 5e-06, 1e-05, 4e-05, 8e-05, .0002, .0005] A  diode_VrMat=[10, 100, 200, 250, 300, 325, 350; 10, 70, 160, 220, 270, 300, 320] V  diode_VrVec=[10, 20, 40, 50, 70, 80, 100] V  diode_IrVec=[1e-06, 2e-06, 5e-06, 1e-05, 2e-05, 5e-05, .0001] A  diode_Vr=-600 V  diode_Ls=150 nH  diode_Erec=0.03 J  diode_rec_loss_model=ee.enum.diode.reverseRecoveryModel.fixed  diode_ErecVal=0 J  diode_scaleWithIandV=true  diode_ErecMat=zeros(2, 3) J  diode_TjrecVec=[298.15, 398.15] K  diode_IfrecVec=[.1, 1, 10] A  diode_IrecVal=10 A  diode_VrecVal=10 V  diode_tFilter=1 / 1000 / 100 s  thermal_network_parameterization=ee.enum.thermalNetworkTopology.external  Rth=[.03, .2] K/W  Rth_Cauer=[.03, .1, .2] K/W  Rth_Foster=[.03, .2] K/W  thermal_mass_parameterization=ee.enum.thermalNetwork.timeconstant  thermal_mass=[3, 25] J/K  thermal_mass_Cauer=[3, 10, 25] J/K  thermal_mass_Foster=[33, 50] J/K  thermal_time_constant=[.1, 5] s  thermal_time_constant_Cauer=[.1, 1, 5] s  thermal_time_constant_Foster=[1, 10] s  thermal_mass_initial_temperatures=[25, 25] degC  thermal_mass_initial_temperatures_Cauer=[25, 25, 25] degC  junction_thermal_mass=0.1 J/K  Tvec_initial_Foster=[25, 25, 25, 25] degC  no_thermal_network=0  junction_temperature_specify=off  junction_temperature_priority=None  junction_temperature=25 degC  junction_temperature_nominal_specify=off  junction_temperature_nominal_value=1  junction_temperature_nominal_unit=degC  Qj_specify=off  Qj_priority=None  Qj=0 W  Qj_nominal_specify=off  Qj_nominal_value=1  Qj_nominal_unit=W  accumulatedSwitchingLosses_specify=off  accumulatedSwitchingLosses_priority=None  accumulatedSwitchingLosses=0 J
  PWM Generator : eePwmGenerator/PWM Generator  CarrCount=Up  Tper=1/10000  Tdelay=0  Ts=0
  Simulink-PS Converter1 : nesl_utility/Simulink-PS Converter  PhysicalDomain=network_engine_domain  SubClassName=ps_input  LeftPortType=input  RightPortType=output  PseudoPeriodic=off  Frequencies=[]  NoiseDistribution=none  NoiseParameters=[]  Unit=V  AffineConversion=off  FilteringAndDerivatives=provide  SimscapeFilterOrder=1  InputFilterTimeConstant=0.001  UdotUserProvided=0
  Step : Step  Time=0.035  After=0  SampleTime=0
  To Workspace : ToWorkspace  VariableName=DC_TFP  SampleTime=-1
  +Term : PMIOPort  Side=Left
  +Out : PMIOPort  Port=2  Side=Right
  -Out : PMIOPort  Port=3  Side=Right
  -Term : PMIOPort  Port=4  Side=Right
  wires:
  Step/1 -> Conversion from percent to decimal/1
  PWM Generator/1 -> Simulink-PS Converter1/1
  Conversion from percent to decimal/1 -> To Workspace/1, PWM Generator/1
  connections:
  Capacitor/LConn1 -- Inductor/RConn1 -- +Out/RConn1
  +Term/RConn1 -- "MOSFET (Ideal, Switching)"/RConn1
  Diode/RConn1 -- "MOSFET (Ideal, Switching)"/RConn2 -- Inductor/LConn1
  Capacitor/RConn1 -- -Term/RConn1 -- Diode/LConn1 -- -Out/RConn1
  "MOSFET (Ideal, Switching)"/LConn1 -- Simulink-PS Converter1/RConn1

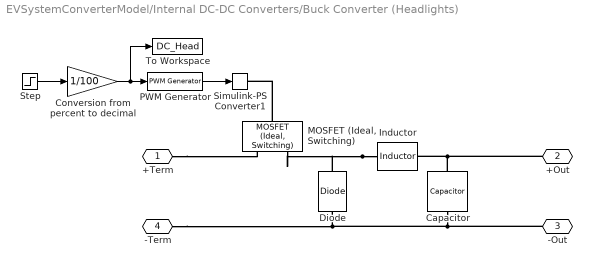
== system EVSystemConverterModel/Internal DC-DC Converters/Buck Converter (Headlights)   ==
  Capacitor : fl_lib/Electrical/Electrical Elements/Capacitor  c=3e-6 F  r=1e-6 Ohm  g=0 1/Ohm  i_specify=off  i_priority=None  i=0 A  i_nominal_specify=off  i_nominal_value=1  i_nominal_unit=A  v_specify=off  v_priority=None  v=0 V  v_nominal_specify=off  v_nominal_value=1  v_nominal_unit=V  vc_specify=off  vc_priority=High  vc=0 V  vc_nominal_specify=off  vc_nominal_value=1  vc_nominal_unit=V
  Conversion from percent to decimal : Gain  Gain=1/100
  Diode : fl_lib/Electrical/Electrical Elements/Diode  Vf=0.6 V  Ron=1e-3 Ohm  Goff=1e-08 1/Ohm  i_specify=off  i_priority=High  i=0 A  i_nominal_specify=off  i_nominal_value=1  i_nominal_unit=A  v_specify=off  v_priority=High  v=0 V  v_nominal_specify=off  v_nominal_value=1  v_nominal_unit=V
  Inductor : fl_lib/Electrical/Electrical Elements/Inductor  l=8e-3 H  r=0 Ohm  g=1e-9 1/Ohm  i_specify=off  i_priority=None  i=0 A  i_nominal_specify=off  i_nominal_value=1  i_nominal_unit=A  v_specify=off  v_priority=None  v=0 V  v_nominal_specify=off  v_nominal_value=1  v_nominal_unit=V  i_L_specify=off  i_L_priority=High  i_L=0 A  i_L_nominal_specify=off  i_L_nominal_value=1  i_L_nominal_unit=A
  "MOSFET (Ideal, Switching)" : ee_lib/Semiconductors & Converters/MOSFET (Ideal, Switching)  port_option=ee.enum.controlport.ps  Rds=1e-3 Ohm  Goff=1e-6 1/Ohm  Vth=0.1 V  diode_param=ee.enum.semiconductors.protectionDiode.external  diode_Vf=0.6 V  diode_Ron=1e-3 Ohm  diode_Goff=1e-5 1/Ohm  diode_C=50e-9 F  diode_iRM=-235 A  diode_iF=300 A  diode_idot=-50 A/us  diode_trr_param=ee.enum.converters.diodeReverseParam.trr_factor  diode_trr_factor=3  diode_trr=15 us  diode_Qrr=1500 s*uA  ids_specify=off  ids_priority=None  ids=0 A  ids_nominal_specify=off  ids_nominal_value=1  ids_nominal_unit=A  vds_specify=off  vds_priority=None  vds=0 V  vds_nominal_specify=off  vds_nominal_value=1  vds_nominal_unit=V  vgs_specify=off  vgs_priority=None  vgs=0 V  vgs_nominal_specify=off  vgs_nominal_value=1  vgs_nominal_unit=V  thermal_loss_option=ee.enum.converters.thermalLossOption.constantvalues  Von_data=[0, 1.8, 3.2, 6, 10, 16; 0, 2, 5.5, 9.5, 15, 25] V  Tj=[298.15, 448.15] K  Iout_data=[0, 20, 40, 60, 80, 100] A  Eon_data=[0, 55.04, 124.57, 235.53, 362.12; 0, 71.25, 161.25, 304.88, 468.75] * 1e-6 J  Eoff_data=[0, 18, 30, 56.1, 76.5; 0, 22.5, 37.5, 70.13, 95.63] * 1e-6 J  Eon_data_3D=[zeros(2, 5, 3)] J  Eoff_data_3D=[zeros(2, 5, 3)] J  Tj_loss=[298.15, 448.15] K  Iout_data_loss=[0, 10, 20, 30, 40] A  tabulateWithVds=false  Vds_loss=[0, 150, 300] V  Eon_scalar=22.86e-3 J  Eoff_scalar=17.14e-3 J  Voff=300 V  Iout_scalar=600 A  useCurrentFromPreviousCycle=false  useVoltageFromPreviousCycle=false  diodeModelType=ee.enum.converters.diodeModelType.pwl  diodeTableType=ee.enum.diode.tableType.IfMat  diode_ReverseIVType=ee.enum.diode.diodeReverseIV.constant  diode_IfMat=[.07, .12, .19, 1.75, 4.24, 7.32, 11.2; .16, .3, .72, 2.14, 4.02, 6.35, 9.12] A  diode_VfMat=[.9, 1.15, 1.25, 1.5, 1.75, 2.17, 2.6, 2.85; .58, .68, .75, 1.1, 1.38, 1.77, 2.27, 2.7] V  diode_TjVec=[25, 125] degC  diode_VfVec=[.5, .7, .9, 1.3, 1.7, 2.1, 2.5] V  diode_IfVec=[.1, .2, .5, 1, 2, 4, 7, 10] A  diode_IrMat=[1e-06, 2e-06, 5e-06, 1e-05, 2.5e-05, 5e-05, .0001; 2e-06, 5e-06, 1e-05, 4e-05, 8e-05, .0002, .0005] A  diode_VrMat=[10, 100, 200, 250, 300, 325, 350; 10, 70, 160, 220, 270, 300, 320] V  diode_VrVec=[10, 20, 40, 50, 70, 80, 100] V  diode_IrVec=[1e-06, 2e-06, 5e-06, 1e-05, 2e-05, 5e-05, .0001] A  diode_Vr=-600 V  diode_Ls=150 nH  diode_Erec=0.03 J  diode_rec_loss_model=ee.enum.diode.reverseRecoveryModel.fixed  diode_ErecVal=0 J  diode_scaleWithIandV=true  diode_ErecMat=zeros(2, 3) J  diode_TjrecVec=[298.15, 398.15] K  diode_IfrecVec=[.1, 1, 10] A  diode_IrecVal=10 A  diode_VrecVal=10 V  diode_tFilter=1 / 1000 / 100 s  thermal_network_parameterization=ee.enum.thermalNetworkTopology.external  Rth=[.03, .2] K/W  Rth_Cauer=[.03, .1, .2] K/W  Rth_Foster=[.03, .2] K/W  thermal_mass_parameterization=ee.enum.thermalNetwork.timeconstant  thermal_mass=[3, 25] J/K  thermal_mass_Cauer=[3, 10, 25] J/K  thermal_mass_Foster=[33, 50] J/K  thermal_time_constant=[.1, 5] s  thermal_time_constant_Cauer=[.1, 1, 5] s  thermal_time_constant_Foster=[1, 10] s  thermal_mass_initial_temperatures=[25, 25] degC  thermal_mass_initial_temperatures_Cauer=[25, 25, 25] degC  junction_thermal_mass=0.1 J/K  Tvec_initial_Foster=[25, 25, 25, 25] degC  no_thermal_network=0  junction_temperature_specify=off  junction_temperature_priority=None  junction_temperature=25 degC  junction_temperature_nominal_specify=off  junction_temperature_nominal_value=1  junction_temperature_nominal_unit=degC  Qj_specify=off  Qj_priority=None  Qj=0 W  Qj_nominal_specify=off  Qj_nominal_value=1  Qj_nominal_unit=W  accumulatedSwitchingLosses_specify=off  accumulatedSwitchingLosses_priority=None  accumulatedSwitchingLosses=0 J
  PWM Generator : eePwmGenerator/PWM Generator  CarrCount=Up  Tper=1/10000  Tdelay=0  Ts=0
  Simulink-PS Converter1 : nesl_utility/Simulink-PS Converter  PhysicalDomain=network_engine_domain  SubClassName=ps_input  LeftPortType=input  RightPortType=output  PseudoPeriodic=off  Frequencies=[]  NoiseDistribution=none  NoiseParameters=[]  Unit=V  AffineConversion=off  FilteringAndDerivatives=provide  SimscapeFilterOrder=1  InputFilterTimeConstant=0.001  UdotUserProvided=0
  Step : Step  Time=0.035  After=0  SampleTime=0
  To Workspace : ToWorkspace  VariableName=DC_Head  SampleTime=-1
  +Term : PMIOPort  Side=Left
  +Out : PMIOPort  Port=2  Side=Right
  -Out : PMIOPort  Port=3  Side=Right
  -Term : PMIOPort  Port=4  Side=Right
  wires:
  PWM Generator/1 -> Simulink-PS Converter1/1
  Step/1 -> Conversion from percent to decimal/1
  Conversion from percent to decimal/1 -> To Workspace/1, PWM Generator/1
  connections:
  "MOSFET (Ideal, Switching)"/LConn1 -- Simulink-PS Converter1/RConn1
  -Out/RConn1 -- Diode/LConn1 -- -Term/RConn1 -- Capacitor/RConn1
  Inductor/LConn1 -- "MOSFET (Ideal, Switching)"/RConn2 -- Diode/RConn1
  +Term/RConn1 -- "MOSFET (Ideal, Switching)"/RConn1
  +Out/RConn1 -- Inductor/RConn1 -- Capacitor/LConn1
